simulink model "Bonis"  (Simulink 7.9)
settings: Solver=ode45  StartTime=0.0  StopTime=10.0  RelTol=1e-3
values from neighbouring files (symbols this model uses):
  A = [0 1 0 ... (first row only)    [ControlOptimo.m]
  b = [0; 0; 1]    [ControlOptimo.m]
  r = 1    [ControlOptimo.m]
  xo = [1;0;0]    [ControlOptimo.m]
settings Model: Creator=satex  LastModifiedBy=satex

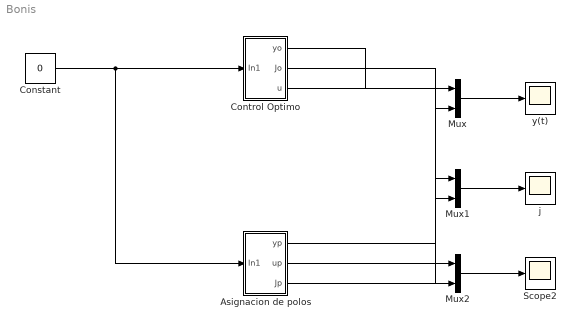
== system Bonis ==
  Asignacion de polos : Subsystem
  Constant : Constant  Value=0
  Control Optimo : Subsystem
  Mux : Mux  Inputs=2
  Mux1 : Mux  Inputs=2
  Mux2 : Mux  Inputs=2
  Scope2 : Scope
      settings: SaveName=ScopeData8
  j : Scope
      settings: SaveName=ScopeData7
  y(t) : Scope
      settings: SaveName=ScopeData6
  wires:
  Mux/1 -> y(t)/1
  Mux1/1 -> j/1
  Mux2/1 -> Scope2/1
  Control Optimo/1(yo) -> Mux/1
  Control Optimo/2(Jo) -> Mux1/1
  Control Optimo/3(u) -> Mux2/1
  Asignacion de polos/1(yp) -> Mux/2
  Asignacion de polos/3(Jp) -> Mux1/2
  Asignacion de polos/2(up) -> Mux2/2
  Constant/1 -> Control Optimo/1(In1), Asignacion de polos/1(In1)

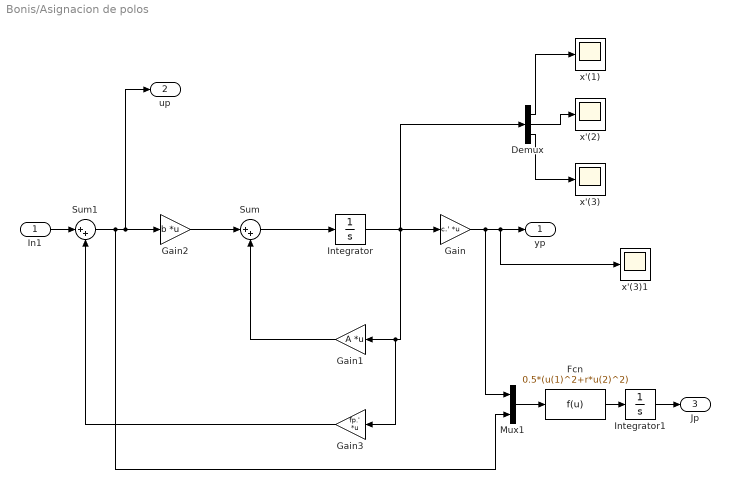
== system Bonis/Asignacion de polos ==
  In1 : Inport
  Demux : Demux  Outputs=3
  Fcn : Fcn  Expr=0.5*(u(1)^2+r*u(2)^2)
  Gain : Gain  Gain=c.'  Multiplication=Matrix(K*u)
  Gain1 : Gain  Gain=A  Multiplication=Matrix(K*u)
  Gain2 : Gain  Gain=b  Multiplication=Matrix(K*u)
  Gain3 : Gain  Gain=fp.'  Multiplication=Matrix(K*u)
  Integrator : Integrator  InitialCondition=xo
  Integrator1 : Integrator
  Mux1 : Mux  Inputs=2
  Sum : Sum  Inputs=|++
  Sum1 : Sum  Inputs=|++
  x'(1) : Scope
      settings: SaveName=ScopeData3
  x'(2) : Scope
      settings: SaveName=ScopeData4
  x'(3) : Scope
      settings: SaveName=ScopeData5
  x'(3)1 : Scope
      settings: SaveName=ScopeData9
  yp : Outport
  up : Outport  Port=2
  Jp : Outport  Port=3
  wires:
  Gain2/1 -> Sum/1
  Gain1/1 -> Sum/2
  Sum/1 -> Integrator/1
  Integrator/1 -> Gain1/1, Gain3/1, Gain/1, Demux/1
  Sum1/1 -> Gain2/1, up/1, Mux1/2
  Gain3/1 -> Sum1/2
  Gain/1 -> Mux1/1, yp/1, x'(3)1/1
  Demux/1 -> x'(1)/1
  Demux/2 -> x'(2)/1
  Demux/3 -> x'(3)/1
  Mux1/1 -> Fcn/1
  Fcn/1 -> Integrator1/1
  In1/1 -> Sum1/1
  Integrator1/1 -> Jp/1

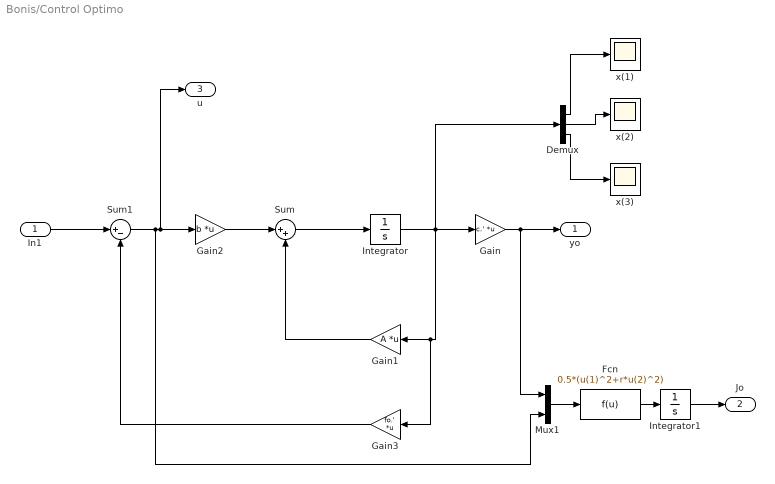
== system Bonis/Control Optimo ==
  In1 : Inport
  Demux : Demux  Outputs=3
  Fcn : Fcn  Expr=0.5*(u(1)^2+r*u(2)^2)
  Gain : Gain  Gain=c.'  Multiplication=Matrix(K*u)
  Gain1 : Gain  Gain=A  Multiplication=Matrix(K*u)
  Gain2 : Gain  Gain=b  Multiplication=Matrix(K*u)
  Gain3 : Gain  Gain=fo.'  Multiplication=Matrix(K*u)
  Integrator : Integrator  InitialCondition=xo
  Integrator1 : Integrator
  Mux1 : Mux  Inputs=2
  Sum : Sum  Inputs=|++
  Sum1 : Sum  Inputs=|+-
  x(1) : Scope
  x(2) : Scope
  x(3) : Scope
      settings: SaveName=ScopeData2
  yo : Outport
  Jo : Outport  Port=2
  u : Outport  Port=3
  wires:
  Sum1/1 -> Mux1/2, Gain2/1, u/1
  Gain3/1 -> Sum1/2
  Gain/1 -> yo/1, Mux1/1
  Demux/1 -> x(1)/1
  Demux/2 -> x(2)/1
  Demux/3 -> x(3)/1
  Integrator1/1 -> Jo/1
  In1/1 -> Sum1/1
  Mux1/1 -> Fcn/1
  Fcn/1 -> Integrator1/1
  Gain2/1 -> Sum/1
  Gain1/1 -> Sum/2
  Sum/1 -> Integrator/1
  Integrator/1 -> Gain1/1, Gain3/1, Gain/1, Demux/1
